simulink model "controle_estabilidade_lqr"  (R2021b)
settings: Solver=ode45  StartTime=0.0  StopTime=100  MaxStep=0.4  RelTol=1e-3
values from neighbouring files (symbols this model uses):
  Bm = 0.0088    [parametros3.mat]    (also in parametros4.mat = 1.398947829e-05)
  Jb = [0.00216966666667  0  0; 0  0.00216966666667  0; 0  0  0.00216966666667]    [parametros3.mat]    (also in parametros4.mat)
  Jm = 0.0015    [parametros2.mat]    (also in parametros3.mat; parametros4.mat = 9.9e-07)
  Jr = 3e-06    [parametros2.mat]    (also in parametros3.mat; parametros4.mat = 9.756e-06)
  K_estab = (LP2_estab*LPL_estab)/1.0    [matlab_script_lead_lag.m]    (also in matlab_script_lqr.m = lqr(A_estab,B_estab,Q_estab,R_estab); matlab_script_lqr_simulink.m = lqr(A_estab,B_estab,Q_estab,R_estab); matlab_script_pd.m = (LP1_estab*LP2_estab*LP3_estab)/LZ1_estab; matlab_script_pd_simulink.m = (LP1_estab*LP2_estab*LP3_estab)/(LZ1_estab*K_tf_forward_esta)
  Kb = 0.000922    [parametros3.mat]    (also in parametros4.mat = 0.02007972426)
  Ki = 0.0264    [parametros3.mat]    (also in parametros4.mat = 0.01969625)
  La = 0.48    [parametros3.mat]    (also in parametros4.mat = 0.0033975)
  Ra = 7    [parametros3.mat]    (also in parametros4.mat = 5.92875)
libraries: sharedutil x2, aerolibutil x2
settings Model: Creator=JRRL  LastModifiedBy=JRRL

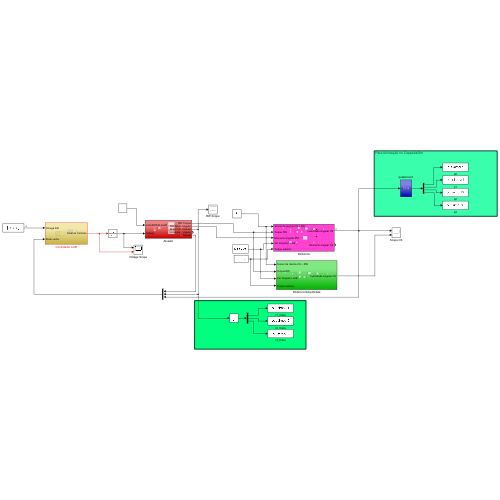
[thumbnail: Simulink's stored preview of the top-level diagram]
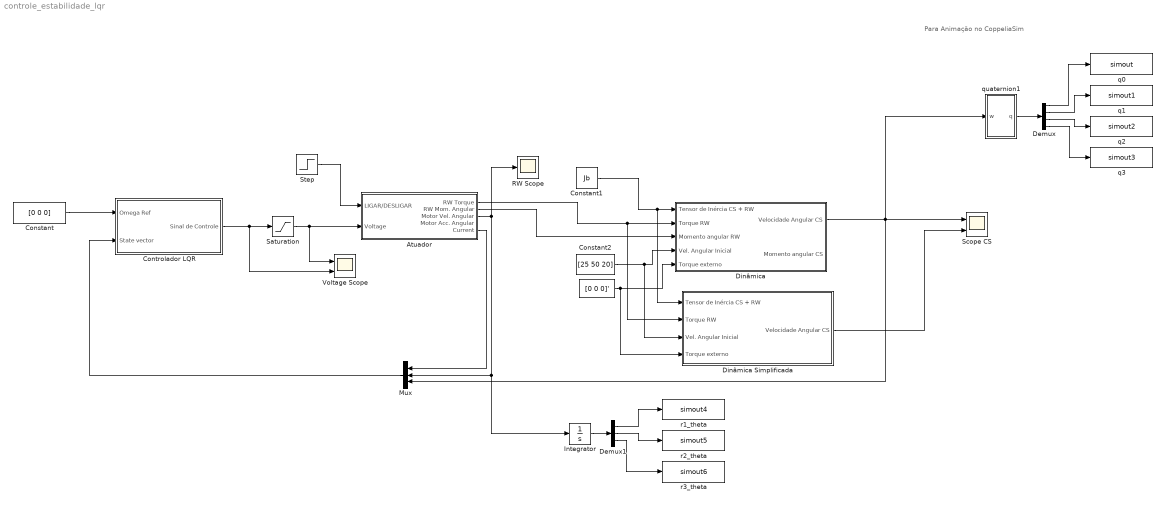
== system controle_estabilidade_lqr ==
  note: Para Animação no CoppeliaSim
  " " : Constant  Value=[0 0 0]'
  Atuador : Subsystem
  Constant : Constant  Value=[0 0 0]
  Constant1 : Constant  Value=Jb
  Constant2 : Constant  Value=[25 50 20]
  Controlador LQR : Subsystem
  Demux : Demux
  Demux1 : Demux  Outputs=3
  Dinâmica : Subsystem
  Dinâmica Simplificada : Subsystem
  Integrator : Integrator
  Mux : Mux  Inputs=3
  RW Scope : Scope
  Saturation : Saturate  UpperLimit=12  LowerLimit=-12
  Scope CS : Scope  NumInputPorts=2
  Step : Step  Time=100  Before=1  SampleTime=0
  Voltage Scope : Scope  NumInputPorts=2
  q0 : ToWorkspace  VariableName=simout  SampleTime=-1
  q1 : ToWorkspace  VariableName=simout1  SampleTime=-1
  q2 : ToWorkspace  VariableName=simout2  SampleTime=-1
  q3 : ToWorkspace  VariableName=simout3  SampleTime=-1
  quaternion1 : Subsystem
  r1_theta : ToWorkspace  VariableName=simout4  SampleTime=-1
  r2_theta : ToWorkspace  VariableName=simout5  SampleTime=-1
  r3_theta : ToWorkspace  VariableName=simout6  SampleTime=-1
  wires:
  Constant1/1 -> Dinâmica Simplificada/1(Tensor de Inércia CS + RW), Dinâmica/1(Tensor de Inércia CS + RW)
  Dinâmica/1(Velocidade Angular CS) -> quaternion1/1(w), Scope CS/1, Mux/3
  Atuador/2(RW Mom. Angular) -> Dinâmica/3(Momento angular RW)
  Constant2/1 -> Dinâmica Simplificada/3(Vel. Angular Inicial), Dinâmica/4(Vel. Angular Inicial)
  " "/1 -> Dinâmica Simplificada/4(Torque externo), Dinâmica/5(Torque externo)
  Atuador/1(RW Torque) -> Dinâmica Simplificada/2(Torque RW), Dinâmica/2(Torque RW)
  Step/1 -> Atuador/1(LIGAR/DESLIGAR)
  Atuador/5(Current) -> Mux/1
  Mux/1 -> Controlador LQR/2(State vector)
  Constant/1 -> Controlador LQR/1(Omega Ref)
  Dinâmica Simplificada/1(Velocidade Angular CS) -> Scope CS/2
  Controlador LQR/1(Sinal de Controle) -> Saturation/1, Voltage Scope/2
  Saturation/1 -> Voltage Scope/1, Atuador/2(Voltage)
  Demux/4 -> q3/1
  Demux/2 -> q1/1
  Demux/3 -> q2/1
  Demux/1 -> q0/1
  quaternion1/1(q) -> Demux/1
  Atuador/3(Motor Vel. Angular) -> RW Scope/1, Integrator/1, Mux/2
  Integrator/1 -> Demux1/1
  Demux1/1 -> r1_theta/1
  Demux1/2 -> r2_theta/1
  Demux1/3 -> r3_theta/1

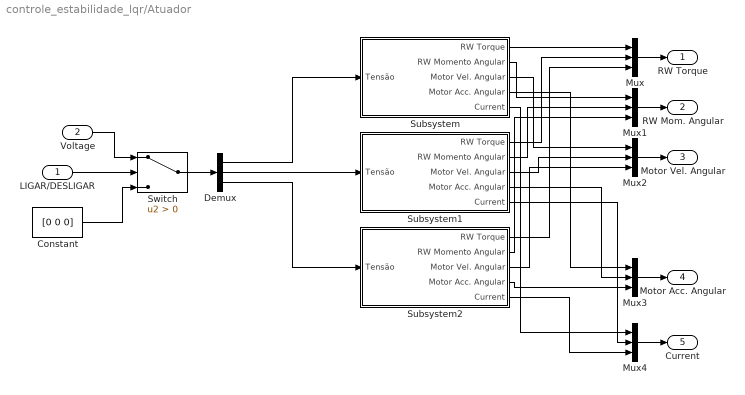
== system controle_estabilidade_lqr/Atuador ==
  LIGAR/DESLIGAR : Inport
  Voltage : Inport  Port=2
  Constant : Constant  Value=[0 0 0]
  Demux : Demux  Outputs=3
  Mux{,1..4} (5 alike) : Mux  Inputs=3
  Subsystem : Subsystem
  Subsystem1 : Subsystem
  Subsystem2 : Subsystem
  Switch : Switch  Criteria=u2 > Threshold
  RW Torque : Outport
  RW Mom. Angular : Outport  Port=2
  Motor Vel. Angular : Outport  Port=3
  Motor Acc. Angular : Outport  Port=4
  Current : Outport  Port=5
  wires:
  Switch/1 -> Demux/1
  Demux/2 -> Subsystem1/1(Tensão)
  Demux/3 -> Subsystem2/1(Tensão)
  Subsystem1/1(RW Torque) -> Mux/2
  Subsystem2/1(RW Torque) -> Mux/3
  Mux/1 -> RW Torque/1
  Mux1/1 -> RW Mom. Angular/1
  Mux2/1 -> Motor Vel. Angular/1
  Mux3/1 -> Motor Acc. Angular/1
  LIGAR/DESLIGAR/1 -> Switch/2
  Voltage/1 -> Switch/1
  Constant/1 -> Switch/3
  Demux/1 -> Subsystem/1(Tensão)
  Subsystem/1(RW Torque) -> Mux/1
  Subsystem/2(RW Momento Angular) -> Mux1/1
  Subsystem/3(Motor Vel. Angular) -> Mux2/1
  Subsystem/4(Motor Acc. Angular) -> Mux3/1
  Mux4/1 -> Current/1
  Subsystem/5(Current) -> Mux4/1
  Subsystem1/2(RW Momento Angular) -> Mux1/2
  Subsystem2/2(RW Momento Angular) -> Mux1/3
  Subsystem1/3(Motor Vel. Angular) -> Mux2/2
  Subsystem2/3(Motor Vel. Angular) -> Mux2/3
  Subsystem1/4(Motor Acc. Angular) -> Mux3/2
  Subsystem2/4(Motor Acc. Angular) -> Mux3/3
  Subsystem1/5(Current) -> Mux4/2
  Subsystem2/5(Current) -> Mux4/3

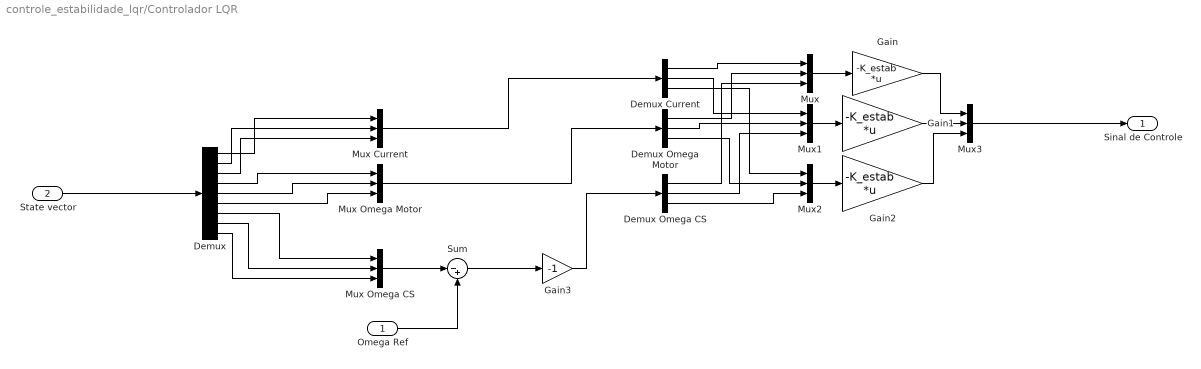
== system controle_estabilidade_lqr/Controlador LQR ==
  Omega Ref : Inport
  State vector : Inport  Port=2
  Demux : Demux  Outputs=9
  Demux Current : Demux  Outputs=3
  Demux Omega CS : Demux  Outputs=3
  Demux Omega Motor : Demux  Outputs=3
  Gain : Gain  Gain=-K_estab  Multiplication=Matrix(K*u)
  Gain1 : Gain  Gain=-K_estab  Multiplication=Matrix(K*u)
  Gain2 : Gain  Gain=-K_estab  Multiplication=Matrix(K*u)
  Gain3 : Gain  Gain=-1
  Mux{,1..3} (4 alike) : Mux  Inputs=3
  Mux Current : Mux  Inputs=3
  Mux Omega CS : Mux  Inputs=3
  Mux Omega Motor : Mux  Inputs=3
  Sum : Sum  Inputs=|-+
  Sinal de Controle : Outport
  wires:
  Mux/1 -> Gain/1
  Mux1/1 -> Gain1/1
  Mux2/1 -> Gain2/1
  Gain1/1 -> Mux3/2
  Gain2/1 -> Mux3/3
  Gain/1 -> Mux3/1
  Mux3/1 -> Sinal de Controle/1
  Demux/1 -> Mux Current/1
  Demux/2 -> Mux Current/2
  Demux/3 -> Mux Current/3
  Demux/5 -> Mux Omega Motor/2
  Demux/6 -> Mux Omega Motor/3
  Demux/4 -> Mux Omega Motor/1
  Mux Current/1 -> Demux Current/1
  Demux Current/1 -> Mux/1
  Demux Current/2 -> Mux1/1
  Demux Current/3 -> Mux2/1
  Demux Omega Motor/1 -> Mux/2
  Demux Omega Motor/2 -> Mux1/2
  Demux Omega Motor/3 -> Mux2/2
  State vector/1 -> Demux/1
  Demux/7 -> Mux Omega CS/1
  Demux/8 -> Mux Omega CS/2
  Demux/9 -> Mux Omega CS/3
  Omega Ref/1 -> Sum/2
  Mux Omega CS/1 -> Sum/1
  Mux Omega Motor/1 -> Demux Omega Motor/1
  Sum/1 -> Gain3/1
  Demux Omega CS/1 -> Mux/3
  Demux Omega CS/2 -> Mux1/3
  Demux Omega CS/3 -> Mux2/3
  Gain3/1 -> Demux Omega CS/1

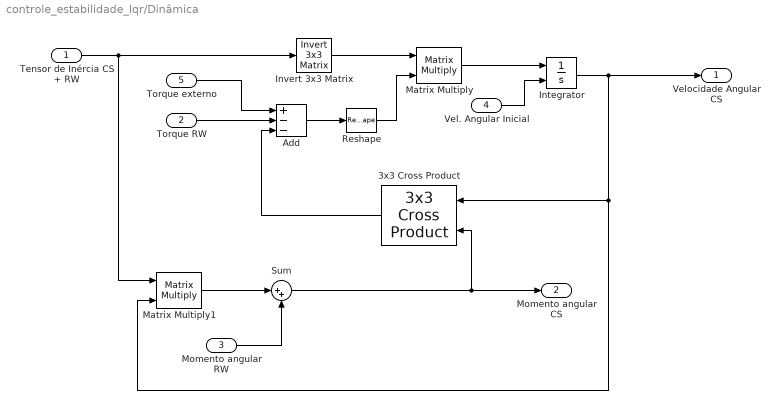
== system controle_estabilidade_lqr/Dinâmica ==
  Tensor de Inércia CS + RW : Inport
  Torque RW : Inport  Port=2
  Momento angular RW : Inport  Port=3
  Vel. Angular Inicial : Inport  Port=4
  Torque externo : Inport  Port=5
  3x3 Cross Product : sharedutil/3x3 Cross Product  aMode=aMode
      settings: SourceProductBaseCode=AE,PW,DR,MT,UV,VE
  Add : Sum  Inputs=+--
  Integrator : Integrator  InitialConditionSource=external
  Invert 3x3 Matrix : aerolibutil/Invert  3x3 Matrix
  Matrix Multiply : Product  Multiplication=Matrix(*)
  Matrix Multiply1 : Product  Multiplication=Matrix(*)
  Reshape : Reshape  OutputDimensionality=Column vector (2-D)
  Sum : Sum  Inputs=|++
  Velocidade Angular CS : Outport
  Momento angular CS : Outport  Port=2
  wires:
  Sum/1 -> Momento angular CS/1, 3x3 Cross Product/2
  3x3 Cross Product/1 -> Add/3
  Invert 3x3 Matrix/1 -> Matrix Multiply/1
  Integrator/1 -> Velocidade Angular CS/1, Matrix Multiply1/2, 3x3 Cross Product/1
  Matrix Multiply/1 -> Integrator/1
  Momento angular RW/1 -> Sum/2
  Torque RW/1 -> Add/2
  Tensor de Inércia CS + RW/1 -> Matrix Multiply1/1, Invert 3x3 Matrix/1
  Torque externo/1 -> Add/1
  Vel. Angular Inicial/1 -> Integrator/2
  Add/1 -> Reshape/1
  Matrix Multiply1/1 -> Sum/1
  Reshape/1 -> Matrix Multiply/2

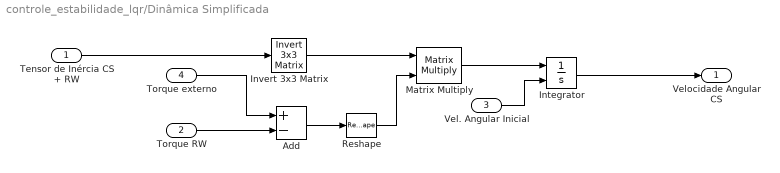
== system controle_estabilidade_lqr/Dinâmica Simplificada ==
  Tensor de Inércia CS + RW : Inport
  Torque RW : Inport  Port=2
  Vel. Angular Inicial : Inport  Port=3
  Torque externo : Inport  Port=4
  Add : Sum  Inputs=+-
  Integrator : Integrator  InitialConditionSource=external
  Invert 3x3 Matrix : aerolibutil/Invert  3x3 Matrix
  Matrix Multiply : Product  Multiplication=Matrix(*)
  Reshape : Reshape  OutputDimensionality=Column vector (2-D)
  Velocidade Angular CS : Outport
  wires:
  Add/1 -> Reshape/1
  Tensor de Inércia CS + RW/1 -> Invert 3x3 Matrix/1
  Torque RW/1 -> Add/2
  Vel. Angular Inicial/1 -> Integrator/2
  Reshape/1 -> Matrix Multiply/2
  Torque externo/1 -> Add/1
  Integrator/1 -> Velocidade Angular CS/1
  Invert 3x3 Matrix/1 -> Matrix Multiply/1
  Matrix Multiply/1 -> Integrator/1

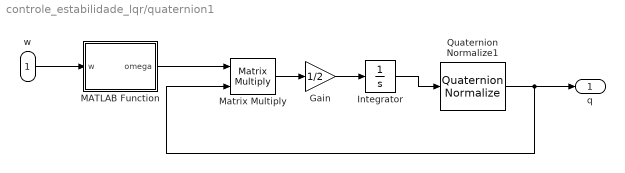
== system controle_estabilidade_lqr/quaternion1 ==
  w : Inport
  Gain : Gain  Gain=1/2
  Integrator : Integrator  InitialCondition=[1 0 0 0]
  MATLAB Function : MATLAB Function  TreatAsAtomicUnit=on
  Matrix Multiply : Product  Multiplication=Matrix(*)
  Quaternion Normalize1 : sharedutil/Quaternion Normalize  aMode=aMode
      settings: SourceProductBaseCode=AE,PW,DR,MT,UV,VE
  q : Outport
  wires:
  w/1 -> MATLAB Function/1(w)
  MATLAB Function/1(omega) -> Matrix Multiply/1
  Quaternion Normalize1/1 -> q/1, Matrix Multiply/2
  Integrator/1 -> Quaternion Normalize1/1
  Gain/1 -> Integrator/1
  Matrix Multiply/1 -> Gain/1

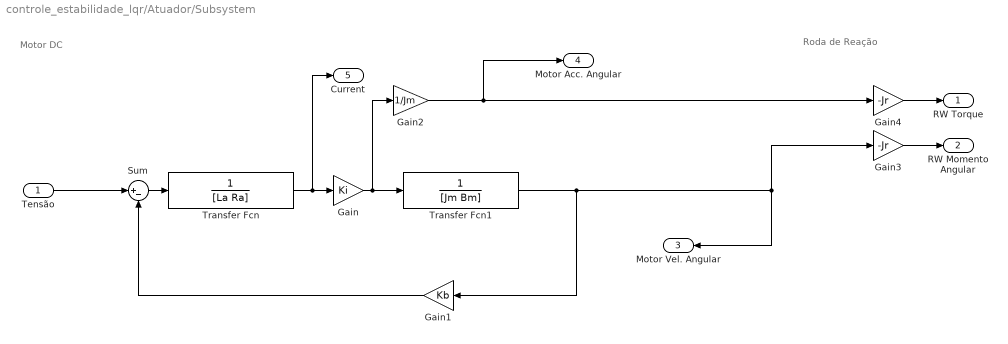
== system controle_estabilidade_lqr/Atuador/Subsystem ==
  note: Roda de Reação
  note: Motor DC
  Tensão : Inport
  Gain : Gain  Gain=Ki
  Gain1 : Gain  Gain=Kb
  Gain2 : Gain  Gain=1/Jm
  Gain3 : Gain  Gain=-Jr
  Gain4 : Gain  Gain=-Jr
  Sum : Sum  Inputs=|+-
  Transfer Fcn : TransferFcn  Denominator=[La Ra]
  Transfer Fcn1 : TransferFcn  Denominator=[Jm Bm]
  RW Torque : Outport
  RW Momento Angular : Outport  Port=2
  Motor Vel. Angular : Outport  Port=3
  Motor Acc. Angular : Outport  Port=4
  Current : Outport  Port=5
  wires:
  Gain/1 -> Transfer Fcn1/1, Gain2/1
  Transfer Fcn/1 -> Current/1, Gain/1
  Gain2/1 -> Gain4/1, Motor Acc. Angular/1
  Transfer Fcn1/1 -> Gain3/1, Motor Vel. Angular/1, Gain1/1
  Sum/1 -> Transfer Fcn/1
  Gain1/1 -> Sum/2
  Gain4/1 -> RW Torque/1
  Tensão/1 -> Sum/1
  Gain3/1 -> RW Momento Angular/1

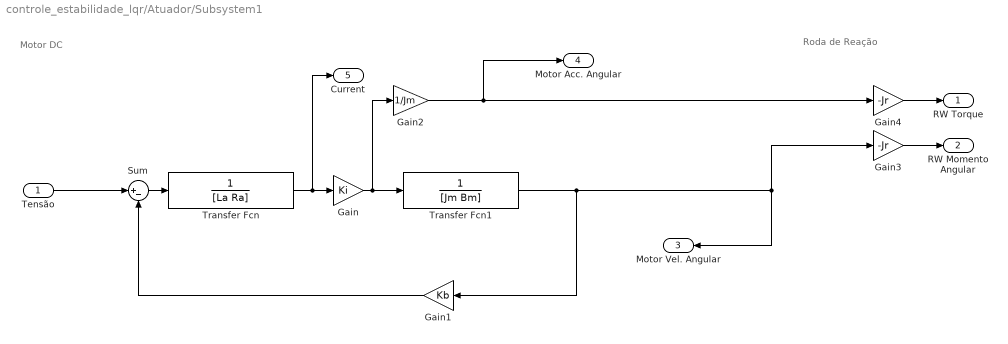
== system controle_estabilidade_lqr/Atuador/Subsystem1 ==
  note: Roda de Reação
  note: Motor DC
  Tensão : Inport
  Gain : Gain  Gain=Ki
  Gain1 : Gain  Gain=Kb
  Gain2 : Gain  Gain=1/Jm
  Gain3 : Gain  Gain=-Jr
  Gain4 : Gain  Gain=-Jr
  Sum : Sum  Inputs=|+-
  Transfer Fcn : TransferFcn  Denominator=[La Ra]
  Transfer Fcn1 : TransferFcn  Denominator=[Jm Bm]
  RW Torque : Outport
  RW Momento Angular : Outport  Port=2
  Motor Vel. Angular : Outport  Port=3
  Motor Acc. Angular : Outport  Port=4
  Current : Outport  Port=5
  wires:
  Gain/1 -> Transfer Fcn1/1, Gain2/1
  Transfer Fcn/1 -> Current/1, Gain/1
  Gain2/1 -> Gain4/1, Motor Acc. Angular/1
  Transfer Fcn1/1 -> Gain3/1, Motor Vel. Angular/1, Gain1/1
  Sum/1 -> Transfer Fcn/1
  Gain1/1 -> Sum/2
  Gain4/1 -> RW Torque/1
  Tensão/1 -> Sum/1
  Gain3/1 -> RW Momento Angular/1

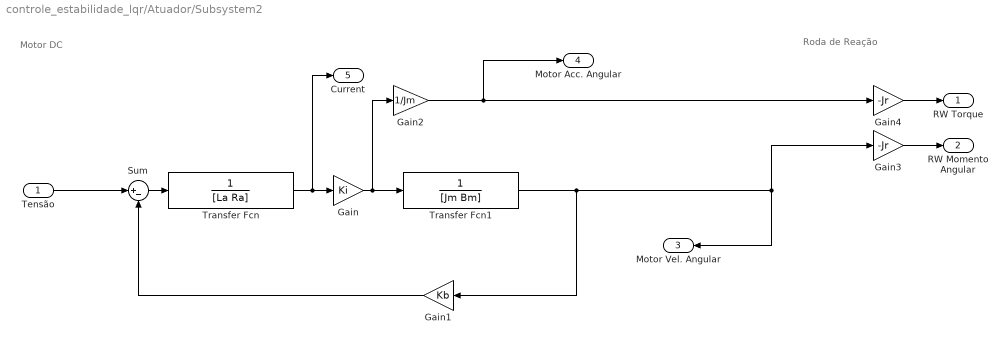
== system controle_estabilidade_lqr/Atuador/Subsystem2 ==
  note: Roda de Reação
  note: Motor DC
  Tensão : Inport
  Gain : Gain  Gain=Ki
  Gain1 : Gain  Gain=Kb
  Gain2 : Gain  Gain=1/Jm
  Gain3 : Gain  Gain=-Jr
  Gain4 : Gain  Gain=-Jr
  Sum : Sum  Inputs=|+-
  Transfer Fcn : TransferFcn  Denominator=[La Ra]
  Transfer Fcn1 : TransferFcn  Denominator=[Jm Bm]
  RW Torque : Outport
  RW Momento Angular : Outport  Port=2
  Motor Vel. Angular : Outport  Port=3
  Motor Acc. Angular : Outport  Port=4
  Current : Outport  Port=5
  wires:
  Gain/1 -> Transfer Fcn1/1, Gain2/1
  Transfer Fcn/1 -> Current/1, Gain/1
  Gain2/1 -> Gain4/1, Motor Acc. Angular/1
  Transfer Fcn1/1 -> Gain3/1, Motor Vel. Angular/1, Gain1/1
  Sum/1 -> Transfer Fcn/1
  Gain1/1 -> Sum/2
  Gain4/1 -> RW Torque/1
  Tensão/1 -> Sum/1
  Gain3/1 -> RW Momento Angular/1

== matlab function controle_estabilidade_lqr/quaternion1/MATLAB Function ==
  data: w input; omega output
function omega = fcn(w)
    wx = w(1);
    wy = w(2);
    wz = w(3);
    res = [0 -wx -wy -wz;wx 0 wz -wy;wy -wz 0 wx;wz wy -wx 0];
omega = res;
